simulink model "Simulink_model"  (R2025b)
settings: Solver=VariableStepAuto  StartTime=0.0  StopTime=10.0  RelTol=1e-3
values from neighbouring files (symbols this model uses):
  rads2rpm = 60/2/pi    (= 9.54929658551)    [Data.m]
undefined symbols (not defined in the file or in its folder): drv, gbox, mld, mot, sens
settings Model: Creator=Enrico  LastModifiedBy=Enrico

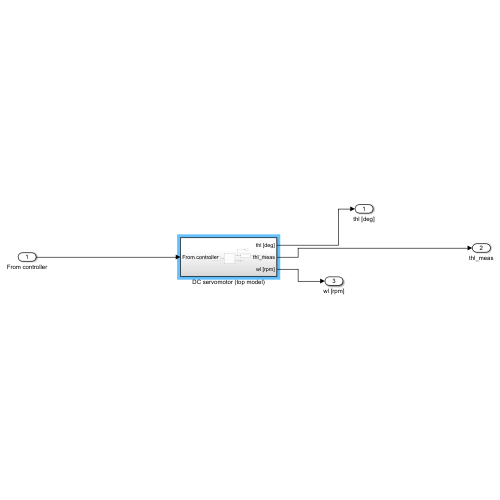
[thumbnail: Simulink's stored preview of the top-level diagram]
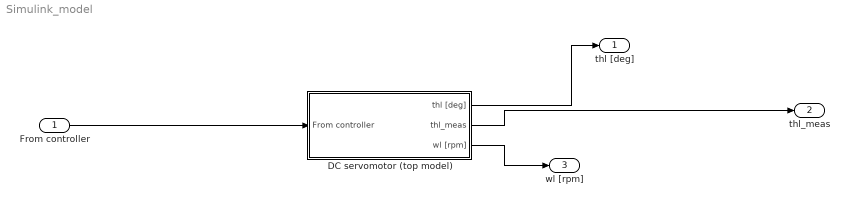
== system Simulink_model ==
  From controller : Inport
  DC servomotor (top model) : Subsystem
  thl [deg] : Outport
  thl_meas : Outport  Port=2
  wl [rpm] : Outport  Port=3
  wires:
  From controller/1 -> DC servomotor (top model)/1(From controller)
  DC servomotor (top model)/1(thl [deg]) -> thl [deg]/1
  DC servomotor (top model)/2(thl_meas) -> thl_meas/1
  DC servomotor (top model)/3(wl [rpm]) -> wl [rpm]/1

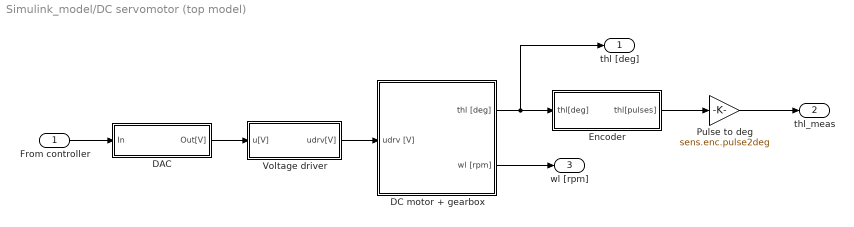
== system Simulink_model/DC servomotor (top model) ==
  From controller : Inport
  DAC : Subsystem
  DC motor + gearbox : Subsystem
  Encoder : Subsystem
  Pulse to deg : Gain  Gain=sens.enc.pulse2deg
  Voltage driver : Subsystem
  thl [deg] : Outport
  thl_meas : Outport  Port=2
  wl [rpm] : Outport  Port=3
  wires:
  Pulse to deg/1 -> thl_meas/1
  DAC/1(Out[V]) -> Voltage driver/1(u[V])
  DC motor + gearbox/2(wl [rpm]) -> wl [rpm]/1
  Voltage driver/1(udrv[V]) -> DC motor + gearbox/1(udrv [V])
  DC motor + gearbox/1(thl [deg]) -> thl [deg]/1, Encoder/1(thl[deg])
  Encoder/1(thl[pulses]) -> Pulse to deg/1
  From controller/1 -> DAC/1(In)

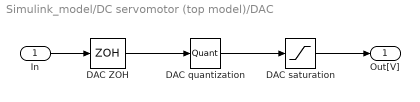
== system Simulink_model/DC servomotor (top model)/DAC ==
  In : Inport
  DAC ZOH : ZeroOrderHold  SampleTime=1e-3
  DAC quantization : Quantizer  QuantizationInterval=20/(2^16 - 1)
  DAC saturation : Saturate  UpperLimit=10  LowerLimit=-10
  Out[V] : Outport
  wires:
  DAC saturation/1 -> Out[V]/1
  DAC ZOH/1 -> DAC quantization/1
  In/1 -> DAC ZOH/1
  DAC quantization/1 -> DAC saturation/1

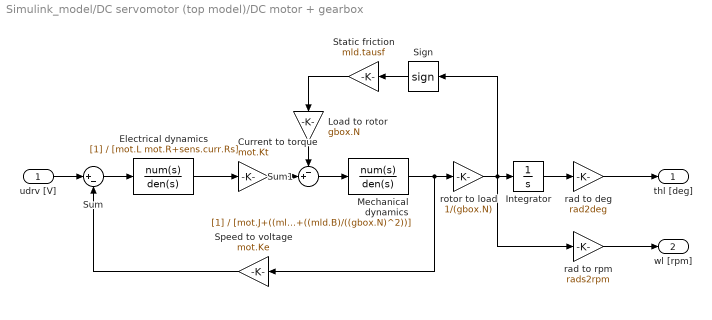
== system Simulink_model/DC servomotor (top model)/DC motor + gearbox ==
  udrv [V] : Inport
  Current to torque : Gain  Gain=mot.Kt
  Electrical dynamics : TransferFcn  Denominator=[mot.L mot.R+sens.curr.Rs]
  Integrator : Integrator
  Load to rotor : Gain  Gain=gbox.N
  Mechanical dynamics : TransferFcn  Denominator=[mot.J+((mld.J)/((gbox.N)^2)) mot.B+((mld.B)/((gbox.N)^2))]
  Sign : Signum
  Speed to voltage : Gain  Gain=mot.Ke
  Static friction : Gain  Gain=mld.tausf
  Sum : Sum  Inputs=|+-
  Sum1 : Sum  Inputs=-+|
  rad to deg : Gain  Gain=rad2deg
  rad to rpm : Gain  Gain=rads2rpm
  rotor to load : Gain  Gain=1/(gbox.N)
  thl [deg] : Outport
  wl [rpm] : Outport  Port=2
  wires:
  Speed to voltage/1 -> Sum/2
  udrv [V]/1 -> Sum/1
  Current to torque/1 -> Sum1/2
  Sum/1 -> Electrical dynamics/1
  Load to rotor/1 -> Sum1/1
  rad to rpm/1 -> wl [rpm]/1
  Mechanical dynamics/1 -> Speed to voltage/1, rotor to load/1
  Electrical dynamics/1 -> Current to torque/1
  rotor to load/1 -> rad to rpm/1, Sign/1, Integrator/1
  Sum1/1 -> Mechanical dynamics/1
  Integrator/1 -> rad to deg/1
  Static friction/1 -> Load to rotor/1
  rad to deg/1 -> thl [deg]/1
  Sign/1 -> Static friction/1

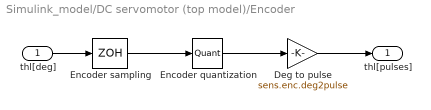
== system Simulink_model/DC servomotor (top model)/Encoder ==
  thl[deg] : Inport
  Deg to pulse : Gain  Gain=sens.enc.deg2pulse
  Encoder quantization : Quantizer
  Encoder sampling : ZeroOrderHold  SampleTime=1e-3
  thl[pulses] : Outport
  wires:
  Deg to pulse/1 -> thl[pulses]/1
  Encoder sampling/1 -> Encoder quantization/1
  thl[deg]/1 -> Encoder sampling/1
  Encoder quantization/1 -> Deg to pulse/1

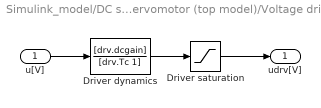
== system Simulink_model/DC servomotor (top model)/Voltage driver ==
  u[V] : Inport
  Driver dynamics : TransferFcn  Numerator=[drv.dcgain]  Denominator=[drv.Tc 1]
  Driver saturation : Saturate  UpperLimit=12  LowerLimit=-12
  udrv[V] : Outport
  wires:
  Driver dynamics/1 -> Driver saturation/1
  Driver saturation/1 -> udrv[V]/1
  u[V]/1 -> Driver dynamics/1
